simulink model "verify_alfa_ceiling_mdl"  (R2018b)
settings: Solver=VariableStepDiscrete  StartTime=0.0  StopTime=10  MaxStep=0.2  RelTol=1e-3  EnableMultiTasking=on
libraries: carnot x2, simulink x1
settings Model: Creator=drhf  LastModifiedBy=drhf
settings DataIOCC: SaveFormat=Array  SignalLoggingSaveFormat=ModelDataLogs
settings OptimizationCC: ExpressionDepthLimit=2147483647  LifeSpan=inf
settings DebuggingCC: UnderspecifiedInitializationDetection=Classic  MergeDetectMultiDrivingBlocksExec=none  SolverPrmCheckMsg=warning  StateNameClashWarn=warning  SFUnexpectedBacktrackingDiag=warning  SFNoUnconditionalDefaultTransitionDiag=warning  SFExecutionAtInitializationDiag=none
settings HardwareCC: ProdBitPerPointer=32  ProdBitPerSizeT=32  ProdBitPerPtrDiffT=32  ProdLargestAtomicFloat=None  ProdIntDivRoundTo=Undefined  ProdEndianess=Unspecified  ProdWordSize=32  ProdHWDeviceType=32-bit Generic
settings ModelReferenceCC: PropagateSignalLabelsOutOfModel=off
settings SFSimCC: SimUseLocalCustomCode=off
settings RTWCC: RTWUseLocalCustomCode=off
settings CodeAppCC: StateflowObjectComments=on
settings GRTTargetCC: TargetLangStandard=C89/C90 (ANSI)  GeneratePreprocessorConditionals=Disable all  CombineOutputUpdateFcns=off  GRTInterface=on
settings ConfigComp: CovMetricSettings=dw  CovHtmlReporting=on  CovSaveCumulativeToWorkspaceVar=on  CovSaveSingleToWorkspaceVar=on  CovExternalEMLEnable=off

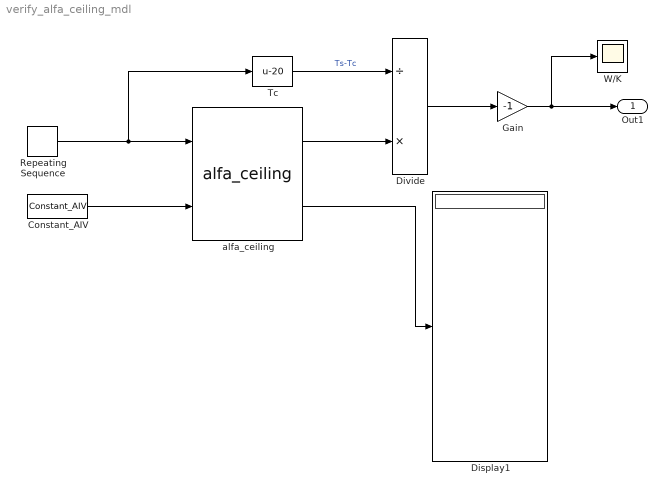
== system verify_alfa_ceiling_mdl ==
  Constant_AIV : carnot/Source/Ventilation/Constant_AIV  Tsens=20  Tcon=20  Trad=20  mw=0.012  mco=0.01  rhoair=1.2  cpair=1004  pair=100000  nair=0.5
  Display1 : Display
  Divide : Product  Inputs=/*
  Gain : Gain  Gain=-1
  Repeating Sequence : simulink/Sources/Repeating Sequence  rep_seq_t=[0 10]  rep_seq_y=[10 30]
  Tc : Bias  Bias=-20
  W/K : Scope
  alfa_ceiling : carnot/Basic/Heat_Transfer/alfa_ceiling  active=0  emission_c=0.65  wallsurface=1
  Out1 : Outport
  wires:
  Gain/1 -> W/K/1, Out1/1
  Constant_AIV/1 -> alfa_ceiling/2
  Repeating Sequence/1 -> Tc/1, alfa_ceiling/1
  Tc/1 -> Divide/1  "Ts-Tc"
  alfa_ceiling/1 -> Divide/2
  Divide/1 -> Gain/1
  alfa_ceiling/2 -> Display1/1
